simulink model "Copy_of_segbot"  (R2021a)
settings: Solver=VariableStepAuto  StartTime=0.0  StopTime=200  RelTol=1e-3
values from neighbouring files (symbols this model uses):
  a = 2*pi*12.5    (= 78.5398163397)    [setbot_more_states.m]    (also in test.m = 235.619449019)
  alpha = (n*K_t)/R_m    (= 0.0488375)    [equations.m]    (also in setbot_more_states.m = 0.208373333333; test.m)
  beta = ((n*K_t*K_b)/R_m) + f_m    (= 0.02128081125)    [equations.m]    (also in setbot_more_states.m = 0.0836114613333; test.m)
  f_m = 0.0022    [equations.m]    (also in setbot_more_states.m; test.m)
  g = 9.81    [equations.m]    (also in setbot_more_states.m; test.m)
  J_m = 2.285e-4    (= 0.0002285)    [equations.m]    (also in setbot_more_states.m; test.m)
  J_psi = (M*L^2)/3    (= 0.00179155878958)    [equations.m]    (also in setbot_more_states.m = 0.000461312133333; test.m = 0.00157383010417)
  J_w = (m*R^2)/2    (= 8.898289e-05)    [equations.m]    (also in setbot_more_states.m = 0.00013803675; test.m)
  K = [-60,-8.8,-3]*12/10    [equations.m]    (also in setbot_more_states.m = place(A,B,[-800,-9,-10,-11]); test.m = lqrd(A,B,Q,R,0.004))
  K_b = 0.3907    [equations.m]    (also in setbot_more_states.m; test.m)
  K_t = 0.3907    [equations.m]    (also in setbot_more_states.m; test.m)
  L = 0.07475    [equations.m]    (also in setbot_more_states.m = 0.049; test.m)
  m = 0.05    [equations.m]    (also in setbot_more_states.m = 0.0615; test.m)
  M = 0.845+0.1169    (= 0.9619)    [equations.m]    (also in setbot_more_states.m = 0.5764; test.m = 0.845)
  n = 1    [equations.m]    (also in setbot_more_states.m; test.m)
  R = 0.05966    [equations.m]    (also in setbot_more_states.m = 0.067; test.m = 0.05)
  R_m = 12/1.5    (= 8)    [equations.m]    (also in setbot_more_states.m = 1.875; test.m)
settings Model: Creator=d-blo  LastModifiedBy=yixia
settings SolverCC: AlgebraicLoopSolver=TrustRegion
settings DataIOCC: ReturnWorkspaceOutputs=off
settings DebuggingCC: SFMachineParentedDataDiag=warning  ArithmeticOperatorsInVariantConditions=warning
settings SFSimCC: CustomCodeUndefinedFunction=UseInterfaceOnly

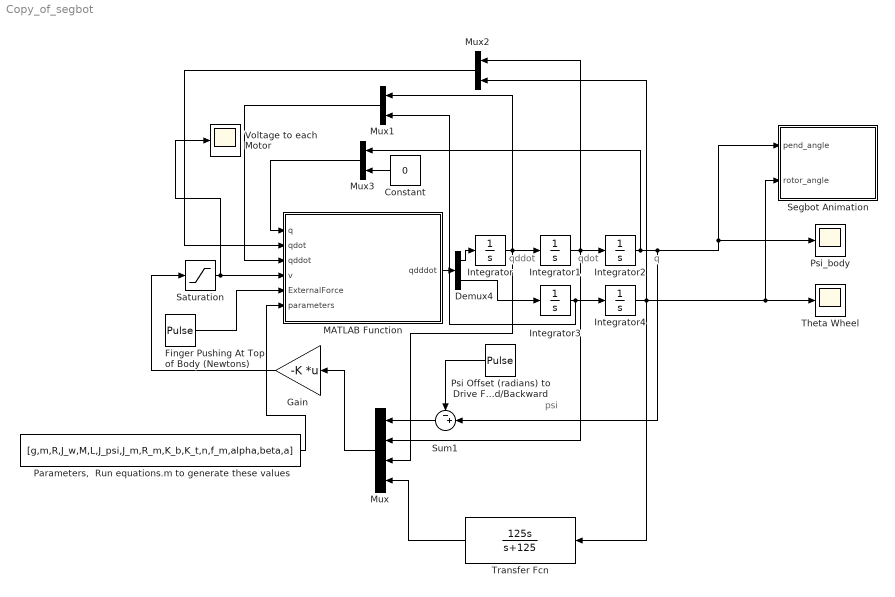
== system Copy_of_segbot ==
  note: psi
  note: qddot
  note: q
  note: qdot
  Constant : Constant  Value=0
  Demux4 : Demux  Outputs=2
  Finger Pushing At Top of Body (Newtons) : DiscretePulseGenerator  PulseType=Time based  Amplitude=0.1  Period=4  PulseWidth=50  PhaseDelay=2
  Gain : Gain  Gain=-K  Multiplication=Matrix(K*u)
  Integrator{,1,3..4} (4 alike) : Integrator
  Integrator2 : Integrator  InitialCondition=0.1
  MATLAB Function : MATLAB Function  TreatAsAtomicUnit=on
  Mux : Mux
  Mux1 : Mux  Inputs=2
  Mux2 : Mux  Inputs=2
  Mux3 : Mux  Inputs=2
  "Parameters,  Run equations.m to generate these values" : Constant  Value=[g,m,R,J_w,M,L,J_psi,J_m,R_m,K_b,K_t,n,f_m,alpha,beta,a]
  Psi Offset (radians) to Drive Forward/Backward : DiscretePulseGenerator  PulseType=Time based  Amplitude=0  Period=4  PulseWidth=50  PhaseDelay=2
  Psi_body : Scope
  Saturation : Saturate  UpperLimit=6  LowerLimit=-6
  Segbot Animation : Subsystem  mask(Segbot Animation){}
      mask help: The animation block takes as input the Segbot body angle (in radians), with 0 straight up and the wheel angle in radians. Use this to visualize the Segbot.
      mask Help: The animation block takes as input the Segbot body angle (in radians), with 0 straight up and the wheel angle in radians.  Use this to visualize the Segbot.
      mask Display:
      | port_label('input', 1, 'Boby Psi')
      | port_label('input', 2, 'Motor Theta')
      | fprintf('Segbot Animation')
  Sum1 : Sum  Inputs=-+|
  Theta Wheel : Scope
  Transfer Fcn : TransferFcn  Numerator=[125 0]  Denominator=[1 125]
  Voltage to each Motor : Scope
  wires:
  MATLAB Function/1(qdddot) -> Demux4/1
  Integrator/1 -> Mux1/1, Integrator1/1, Mux/3
  Mux/1 -> Gain/1
  Integrator2/1 -> Mux3/1, Sum1/2, Segbot Animation/1(pend_angle), Psi_body/1
  Gain/1 -> Saturation/1
  Saturation/1 -> Voltage to each Motor/1, MATLAB Function/4(v)
  Psi Offset (radians) to Drive Forward/Backward/1 -> Sum1/1
  Sum1/1 -> Mux/1
  "Parameters,  Run equations.m to generate these values"/1 -> MATLAB Function/6(parameters)
  Finger Pushing At Top of Body (Newtons)/1 -> MATLAB Function/5(ExternalForce)
  Transfer Fcn/1 -> Mux/4
  Integrator1/1 -> Mux2/1, Integrator2/1, Mux/2
  Integrator3/1 -> Mux1/2, Integrator4/1
  Demux4/1 -> Integrator/1
  Demux4/2 -> Integrator3/1
  Integrator4/1 -> Mux2/2, Segbot Animation/2(rotor_angle), Theta Wheel/1, Transfer Fcn/1
  Mux1/1 -> MATLAB Function/3(qddot)
  Mux2/1 -> MATLAB Function/2(qdot)
  Mux3/1 -> MATLAB Function/1(q)
  Constant/1 -> Mux3/2

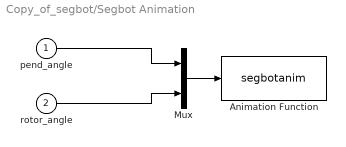
== system Copy_of_segbot/Segbot Animation ==
  pend_angle : Inport
  rotor_angle : Inport  Port=2
  Animation Function : S-Function  FunctionName=segbotanim  Parameters=0.05  SFunctionDeploymentMode=off  EnableBusSupport=off
      settings: DeleteFcn=if ~isempty(findobj('type','figure','name','dblpend1 Animation'));close('dblpend1 Animation'); end;
  Mux : Mux  Inputs=2
  wires:
  Mux/1 -> Animation Function/1
  rotor_angle/1 -> Mux/2
  pend_angle/1 -> Mux/1

== matlab function Copy_of_segbot/MATLAB Function ==
  data: q input; qdddot output; qdot input; qddot input; v input; ExternalForce input; parameters input
function qdddot = fcn(q,qdot,qddot,v,ExternalForce,parameters)

% These are the parameters for the Lego NXTway.
% g = 9.81;
% m = 0.03;
% R = 0.04;
% J_w = (m*R^2)/2;
% M = 0.6;
% L = 0.144/2;
% J_psi = (M*L^2)/3;
% J_m = 1e-5;
% R_m = 6.69;
% K_b = 0.468;
% K_t = 0.317;
% n = 1;
% f_m = 0.0022;
% alpha = (n*K_t)/R_m;
% beta = ((n*K_t*K_b)/R_m) + f_m;

% input parameters so that you can change them in the Matlab command window
% and then they are used in your simulation.
g = parameters(1);
m = parameters(2);
R = parameters(3);
J_w = parameters(4);
M = parameters(5);
L = parameters(6);
J_psi = parameters(7);
J_m = parameters(8);
R_m = parameters(9);
K_b = parameters(10);
K_t = parameters(11);
n = parameters(12);
f_m = parameters(13);
alpha = parameters(14);
beta = parameters(15);
a = parameters(16);

psi = q(1);
psi_d = qdot(1);
psi_dd = qddot(1);
theta_d = qdot(2);

psi_a = psi_d/a-psi;
psi_da = psi_dd/a-psi_d;

D = [(M*L^2 + J_psi + 2*n^2*J_m) (M*L*R*cos(psi_a) - 2*n^2*J_m);
    (M*L*R*cos(psi_a) - 2*n^2*J_m) ((2*m+M)*R^2 + 2*J_w + 2*n^2*J_m)];

h = [M*g*L*sin(psi_a) - 2*beta*psi_da + 2*beta*theta_d - 2*alpha*v + ExternalForce*L*2;
    M*L*R*(psi_da^2)*sin(psi_a) + 2*beta*psi_da - 2*beta*theta_d + 2*alpha*v];

qdddot = (D)\h;
qdddot(1) = a*(qdddot(1)+psi_dd)
